simulink model "InitialDisplacement_TestModel"  (R2014a)
settings: Solver=ode45  StartTime=0.0  StopTime=10.0  RelTol=1e-3
libraries: rocket_angular_flight_library x1
settings Model: Creator=scorpii  LastModifiedBy=scorpii

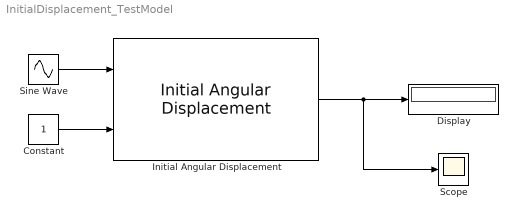
== system InitialDisplacement_TestModel ==
  Constant : Constant
  Display : Display
  Initial Angular Displacement : rocket_angular_flight_library/Initial Angular Displacement
  Scope : Scope
  Sine Wave : Sin  SampleTime=0
  wires:
  Sine Wave/1 -> Initial Angular Displacement/1
  Constant/1 -> Initial Angular Displacement/2
  Initial Angular Displacement/1 -> Scope/1, Display/1
